simulink model "rasoc_tesis_v4"  (R2021a)
settings: Solver=FixedStepAuto  StartTime=0.0  StopTime=inf  FixedStep=0.01  RelTol=1e-3
values from neighbouring files (symbols this model uses):
  a = 0.445    [param_tesis.m]
  a_max = v_max/dt    (= 0.8)    [param_tesis.m]
  alt_z = 0    [param_tesis.m]
  B = 0.5    [param_tesis.m]
  currentPose = [47 43.5 0]    [param_tesis.m]
  efic_red = 0.95    [param_tesis.m]
  goalPose = [1.5 5 pi/2]    [param_tesis.m]
  gpsBasePose = [1 44]    [param_tesis.m]
  kb = 8.93*(3/(1000*pi))    (= 0.00852752185086)    [param_tesis.m]
  kt = 0.077*sqrt(2)*3    [param_tesis.m]
  L = 0.55    [param_tesis.m]
  m_uva = 0    [param_tesis.m]
  n = 16    [param_tesis.m]
  r = 0.125    [param_tesis.m]
  Ra = Vnom/Ipeak    (= 14.2857142857)    [param_tesis.m]
  Rp = Ra*20    (= 285.714285714)    [param_tesis.m]
  t_lpf = 1/200    (= 0.005)    [param_tesis.m]
  tau_max = 5    [param_tesis.m]
  v_max = 0.8    [param_tesis.m]
  Vnom = 310    [param_tesis.m]
  w_max = 0.5    [param_tesis.m]
  waypoints = [currentPose(1), currentPose(2) ... (first row only)    [AstarHybrid_fn.m]    (also in param_tesis.m = AstarHybrid_fn(currentPose, goalPose))
undefined symbols (not defined in the file or in its folder): angular, DiscIntNeverNeededParam, Earth, linear, startTheta, startX, startY, WGS84
libraries: ros2lib x10, simulink x5, mobileRoboticsTrainingLib x3, robotmobilelib x2, pid_lib x2, robotalgslib x2, aerolibtransform2 x2, dspstat3 x1
(part 1 of 2)
settings Model: PacingRate=0.500000  OrderedModelArguments=off  Creator=maxim  LastModifiedBy=maxim
settings DataIOCC: InspectSignalLogs=on
settings OptimizationCC: DefaultParameterBehavior=Inlined  EnhancedBackFolding=on  PassReuseOutputArgsAs=Individual arguments  ZeroExternalMemoryAtStartup=off  ZeroInternalMemoryAtStartup=off  MaxStackSize=64  OptimizeBlockOrder=speed  DifferentSizesBufferReuse=on  OptimizationCustomize=off  EfficientTunableParamExpr=on
settings DebuggingCC: ParameterTunabilityLossMsg=error  SFMachineParentedDataDiag=warning
settings SFSimCC: MATLABDynamicMemAlloc=off
settings RTWCC: SystemTargetFile=ert.tlc  TemplateMakefile=ert_default_tmf  Toolchain=Colcon Tools
settings CodeAppCC: ForceParamTrailComments=on  IgnoreCustomStorageClasses=off  OperatorAnnotations=on  SimulinkDataObjDesc=on  SFDataObjDesc=on  InsertBlockDesc=on
settings ERTTargetCC: RootIOFormat=Structure reference  ERTCustomFileTemplate=example_file_process.tlc

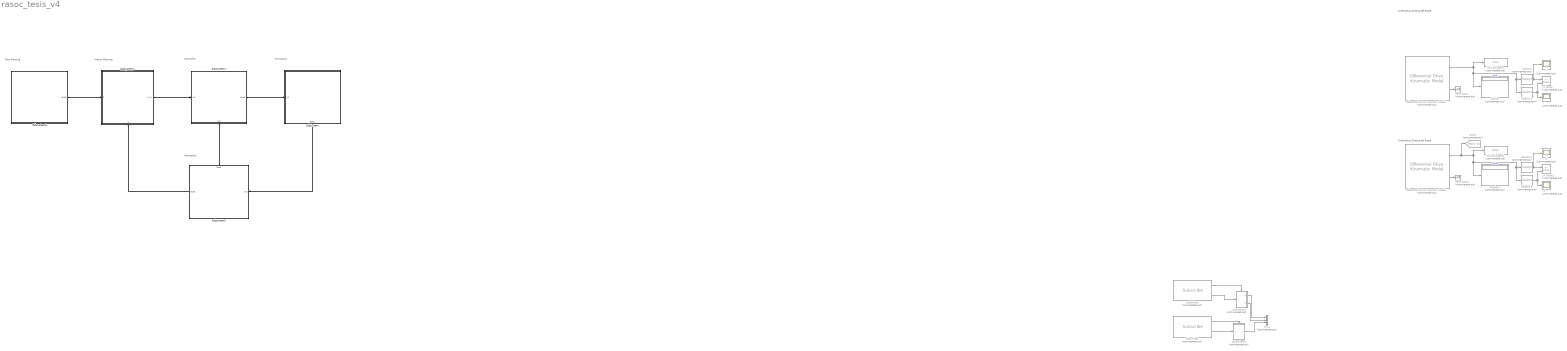
== system rasoc_tesis_v4 ==
  note: Cinemática Directa del Robot
  note: Motion Planning
  note: Controller
  note: Cinemática Directa del Robot
  note: Simulation
  note: Perception
  note: Path Planning
  Differential Drive Kinematic Model1 : robotmobilelib/Differential Drive Kinematic Model  Commented=on  VehicleInputs=Wheel Speeds  WheelRadius=r  WheelSpeedRange=[-inf inf]  TrackWidth=L  InitialState=[currentPose]'  SimulateUsing=Interpreted execution
      settings: SourceProductBaseCode=RO
  Differential Drive Kinematic Model2 : robotmobilelib/Differential Drive Kinematic Model  Commented=on  VehicleInputs=Vehicle Speed & Heading Angular Velocity  WheelRadius=r  WheelSpeedRange=[-inf inf]  TrackWidth=L  InitialState=[currentPose]'  SimulateUsing=Interpreted execution
      settings: SourceProductBaseCode=RO
  Display : Display  Commented=on
  Display1 : Display  Commented=on
  Goto4 : Goto  Commented=on  GotoTag=Pose_ros
  Mux1 : Mux  Commented=on  Inputs=3
  Selector : Selector  Commented=on  InputPortWidth=3  IndexOptions=Index vector (dialog)  Indices=[1]  OutputSizes=1
  Selector1 : Selector  Commented=on  InputPortWidth=3  IndexOptions=Index vector (dialog)  Indices=[2]  OutputSizes=1
  Selector2 : Selector  Commented=on  InputPortWidth=3  IndexOptions=Index vector (dialog)  Indices=[1]  OutputSizes=1
  Selector3 : Selector  Commented=on  InputPortWidth=3  IndexOptions=Index vector (dialog)  Indices=[2]  OutputSizes=1
  Subscribe1 : ros2lib/Subscribe  Commented=on  topicSource=Select from ROS network  topic=/odom  messageType=nav_msgs/Odometry  sampleTime=-1  QOSHistory=Keep last  QOSDepth=1  QOSReliability=Reliable  QOSDurability=Volatile
      settings: SourceProductBaseCode=RR
  Subscribe2 : ros2lib/Subscribe  Commented=on  topicSource=Select from ROS network  topic=/imu  messageType=sensor_msgs/Imu  sampleTime=-1  QOSHistory=Keep last  QOSDepth=1  QOSReliability=Reliable  QOSDurability=Volatile
      settings: SourceProductBaseCode=RR
  Subsystem : Subsystem
      settings: PortSchema="{\"entries\":[{\"content\":{\"sides\":[{\"content\":{\"connectorIds\":[\"In1\"]},\"type\":\"ConnectorPlacement.EquallySpacedRectSide\",\"uuid\":\"273e7eb3-3d1c-4843-aace-07e5779ada44\"},{\"content\":{\"connectorIds\":[],\"side\":\"RIGHT\"},\"type\":\"ConnectorPlacement.EquallySpacedRectSide\",\"uuid\":\"0ce8f36d-1762-4e21-817b-fb4bacc71d23\"},{\"content\":{\"connectorIds\":[],\"side\":\"TOP\"},\"type\":\"ConnectorPlacement.EquallySpacedRectSide\",\"uuid\":\"ca3ae62e-f410-42bb-944a-1dc9a9a102f7\"},{\"content\":{\"connectorIds\":[\"Out1\"],\"side\":\"BOTTOM\"},\"type\":\"ConnectorPlacement.EquallySpacedRectSide\",\"uuid\":\"b5aea1c3-8e14-4876-abba-3cc2b9e42095\"}]},\"type\":\"ConnectorPlacement.EquallySpacedConnector\",\"uuid\":\"a568fb3c-eb3c-49ee-882f-7e9a9c244b7d\"}],\"packageUris\":[\"http://schema.mathworks.com/mf0/Connector/R2020b\"],\"version\":\"1.0\"}"
      mask Display: image('$imagefile'); % Use "Edit Image" on toolstrip to change.
  Subsystem1 : Subsystem
      settings: PortSchema="{\"entries\":[{\"content\":{\"sides\":[{\"content\":{\"connectorIds\":[\"In1\"]},\"type\":\"ConnectorPlacement.EquallySpacedRectSide\",\"uuid\":\"7cc506d6-0df9-4dcf-87be-1a8fc33368cf\"},{\"content\":{\"connectorIds\":[\"Out1\"],\"side\":\"RIGHT\"},\"type\":\"ConnectorPlacement.EquallySpacedRectSide\",\"uuid\":\"9bee288a-7334-4d77-9b50-8b8395b9bab7\"},{\"content\":{\"connectorIds\":[],\"side\":\"TOP\"},\"type\":\"ConnectorPlacement.EquallySpacedRectSide\",\"uuid\":\"546aa84f-61a2-494c-9877-240dac3c06f9\"},{\"content\":{\"connectorIds\":[\"In2\"],\"side\":\"BOTTOM\"},\"type\":\"ConnectorPlacement.EquallySpacedRectSide\",\"uuid\":\"7e0fe68b-13b1-4e4e-82a9-96ee51fb6404\"}]},\"type\":\"ConnectorPlacement.EquallySpacedConnector\",\"uuid\":\"3eddb344-86cd-457c-a24d-297fc14890b0\"}],\"packageUris\":[\"http://schema.mathworks.com/mf0/Connector/R2020b\"],\"version\":\"1.0\"}"
      mask Display: image('$imagefile'); % Use "Edit Image" on toolstrip to change.
  Subsystem2 : Subsystem  Commented=on
  Subsystem3 : Subsystem  Commented=on
  Subsystem4 : Subsystem
      settings: PortSchema="{\"entries\":[{\"content\":{\"sides\":[{\"content\":{\"connectorIds\":[\"In1\"]},\"type\":\"ConnectorPlacement.EquallySpacedRectSide\",\"uuid\":\"4026ad61-f4ec-4a91-9be9-057f2d314736\"},{\"content\":{\"connectorIds\":[\"Out1\"],\"side\":\"RIGHT\"},\"type\":\"ConnectorPlacement.EquallySpacedRectSide\",\"uuid\":\"7c96fecf-2a17-4edc-9dde-8c00b1d53d18\"},{\"content\":{\"connectorIds\":[],\"side\":\"TOP\"},\"type\":\"ConnectorPlacement.EquallySpacedRectSide\",\"uuid\":\"976d1fbd-e5db-4716-a28c-2d13b9cfe893\"},{\"content\":{\"connectorIds\":[\"In2\"],\"side\":\"BOTTOM\"},\"type\":\"ConnectorPlacement.EquallySpacedRectSide\",\"uuid\":\"ea9d66a8-6726-4d07-bc02-8beb6f695a87\"}]},\"type\":\"ConnectorPlacement.EquallySpacedConnector\",\"uuid\":\"2f53d576-4576-48b6-bcca-625d1da1addb\"}],\"packageUris\":[\"http://schema.mathworks.com/mf0/Connector/R2020b\"],\"version\":\"1.0\"}"
      mask Display: image('$imagefile'); % Use "Edit Image" on toolstrip to change.
  Subsystem5 : Subsystem
      settings: PortSchema="{\"entries\":[{\"content\":{\"sides\":[{\"content\":{\"connectorIds\":[\"Out2\"]},\"type\":\"ConnectorPlacement.EquallySpacedRectSide\",\"uuid\":\"c37bb481-eb7e-4f76-88a9-7f2083741892\"},{\"content\":{\"connectorIds\":[\"In1\"],\"side\":\"RIGHT\"},\"type\":\"ConnectorPlacement.EquallySpacedRectSide\",\"uuid\":\"486068a6-059f-443b-b346-93df6811aae6\"},{\"content\":{\"connectorIds\":[\"Out1\"],\"side\":\"TOP\"},\"type\":\"ConnectorPlacement.EquallySpacedRectSide\",\"uuid\":\"f054f05a-6c52-4114-8c0f-0faeb4030005\"}]},\"type\":\"ConnectorPlacement.EquallySpacedConnector\",\"uuid\":\"e0be5d63-417f-4805-bb33-2fed0a69e720\"}],\"packageUris\":[\"http://schema.mathworks.com/mf0/Connector/R2020b\"],\"version\":\"1.0\"}"
      mask Display: image('$imagefile'); % Use "Edit Image" on toolstrip to change.
  Subsystem6 : Subsystem
      mask Display: image('$imagefile'); % Use "Edit Image" on toolstrip to change.
  Terminator : Terminator  Commented=on
  Terminator1 : Terminator  Commented=on
  To Workspace : ToWorkspace  Commented=on  VariableName=Pose  SampleTime=-1
  To Workspace1 : ToWorkspace  Commented=on  VariableName=Pose1  SampleTime=-1
  XY Graph : simulink/Sinks/XY Graph  Commented=on  xmin=0  xmax=50  ymin=-5  ymax=40  st=-1
  XY Graph1 : simulink/Sinks/XY Graph  Commented=on  xmin=0  xmax=25  ymin=0  ymax=25  st=-1
  x : Scope  Commented=on
  x1 : Scope  Commented=on
  y : Scope  Commented=on
  y1 : Scope  Commented=on
  wires:
  Differential Drive Kinematic Model1/1 -> To Workspace/1, Selector1/1, Selector/1, Display/1  "state"
  Selector1/1 -> y/1, XY Graph/2
  Selector/1 -> x/1, XY Graph/1
  Differential Drive Kinematic Model1/2 -> Terminator/1
  Differential Drive Kinematic Model2/2 -> Terminator1/1
  Selector2/1 -> XY Graph1/1, x1/1
  Selector3/1 -> XY Graph1/2, y1/1
  Differential Drive Kinematic Model2/1 -> Goto4/1, Display1/1, Selector2/1, Selector3/1, To Workspace1/1  "state"
  Subsystem2/1(x_ros) -> Mux1/1
  Subscribe2/1 -> Subsystem3/Enable
  Subscribe1/1 -> Subsystem2/Enable
  Subscribe1/2 -> Subsystem2/1(In1)
  Subsystem2/2(y_ros) -> Mux1/2
  Subsystem3/1(angZ_ros) -> Mux1/3
  Subscribe2/2 -> Subsystem3/1(In1)
  Subsystem4/1(v* w*) -> Subsystem1/1(In1)
  Subsystem1/1(Out1) -> Subsystem/1(In1)
  Subsystem/1(Out1) -> Subsystem5/1(In1)
  Subsystem5/2(Out1) -> Subsystem4/2(2)
  Subsystem6/1(Out1) -> Subsystem4/1(1)
  Subsystem5/1(Out2) -> Subsystem1/2(In2)

== system rasoc_tesis_v4/Subsystem ==
  note: wL
  note: wR
  In1 : Inport
  Bus Selector1 : BusSelector  OutputSignals=wL,wR
  OutputROSGazebo : Subsystem
  Out1 : Outport
  wires:
  [newMsg] -> OutputROSGazebo/Enable
  Bus Selector1/2 -> OutputROSGazebo/3(wR)  "<wR>"
  [atGoal] -> OutputROSGazebo/1(atGoal)
  Bus Selector1/1 -> OutputROSGazebo/2(wL)  "<wL>"
  In1/1 -> Bus Selector1/1

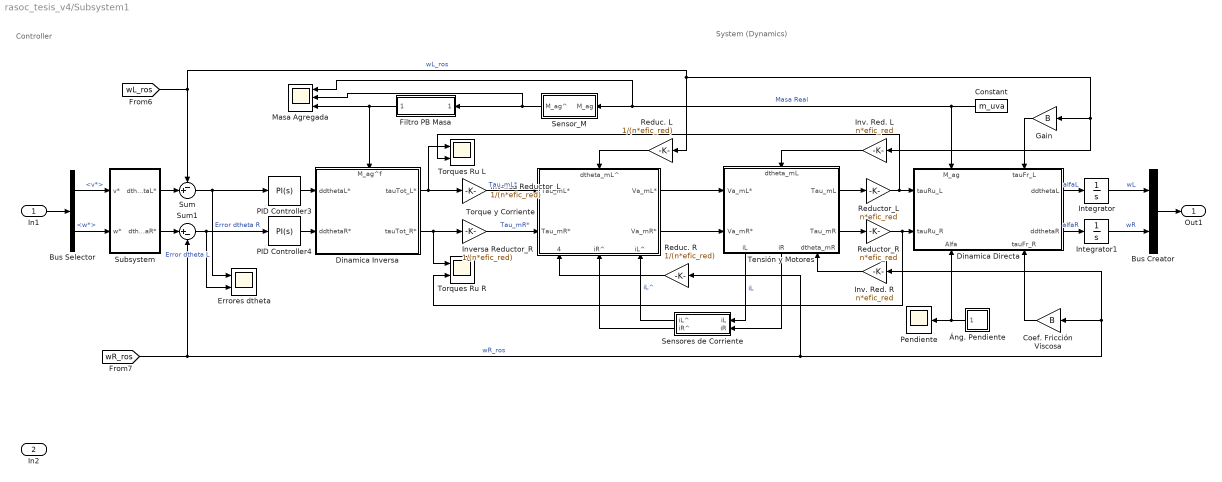
== system rasoc_tesis_v4/Subsystem1 ==
  note: Controller
  note: System (Dynamics)
  In1 : Inport
  In2 : Inport  Port=2
  Bus Creator : BusCreator  Inputs=2
  Bus Selector : BusSelector  OutputSignals=v*,w*
  Coef. Fricción Viscosa : Gain  Gain=B
  Constant : Constant  Value=m_uva
  Dinamica Directa : Subsystem
      settings: PortSchema="{\"entries\":[{\"content\":{\"sides\":[{\"content\":{\"connectorIds\":[\"In1\",\"In2\"]},\"type\":\"ConnectorPlacement.EquallySpacedRectSide\",\"uuid\":\"7724baec-8741-4c83-ab66-71b62264b439\"},{\"content\":{\"connectorIds\":[\"Out1\",\"Out2\"],\"side\":\"RIGHT\"},\"type\":\"ConnectorPlacement.EquallySpacedRectSide\",\"uuid\":\"83de1d79-8442-4360-ae36-8e267c42d9e7\"},{\"content\":{\"connectorIds\":[\"In3\",\"In4\"],\"side\":\"TOP\"},\"type\":\"ConnectorPlacement.EquallySpacedRectSide\",\"uuid\":\"5aa5624d-c3b7-443e-8b1c-4062683451e9\"},{\"content\":{\"connectorIds\":[\"In5\",\"In6\"],\"side\":\"BOTTOM\"},\"type\":\"ConnectorPlacement.EquallySpacedRectSide\",\"uuid\":\"38a03690-6302-43f4-ab4b-44458b1dd3d1\"}]},\"type\":\"ConnectorPlacement.EquallySpacedConnector\",\"uuid\":\"796ba574-cbe1-4118-90ae-27198d609312\"}],\"packageUris\":[\"http://schema.mathworks.com/mf0/Connector/R2020b\"],\"version\":\"1.0\"}"
  Dinamica Inversa : Subsystem
      settings: PortSchema="{\"entries\":[{\"content\":{\"sides\":[{\"content\":{\"connectorIds\":[\"In1\",\"In2\"]},\"type\":\"ConnectorPlacement.EquallySpacedRectSide\",\"uuid\":\"0faee1a4-a132-48bd-bc38-20a06c869d2e\"},{\"content\":{\"connectorIds\":[\"Out1\",\"Out2\"],\"side\":\"RIGHT\"},\"type\":\"ConnectorPlacement.EquallySpacedRectSide\",\"uuid\":\"c1af3771-28d7-4ef6-a87a-ceeaee1edff6\"},{\"content\":{\"connectorIds\":[\"In3\"],\"side\":\"TOP\"},\"type\":\"ConnectorPlacement.EquallySpacedRectSide\",\"uuid\":\"b4509dad-c3f6-4e9a-919d-cf82e4bac41d\"}]},\"type\":\"ConnectorPlacement.EquallySpacedConnector\",\"uuid\":\"1e7b5fad-e8ed-45a7-be76-1d23f7a948ab\"}],\"packageUris\":[\"http://schema.mathworks.com/mf0/Connector/R2020b\"],\"version\":\"1.0\"}"
  Errores dtheta : Scope  NumInputPorts=2
  Filtro PB Masa : Subsystem
  Gain : Gain  Gain=B
  Integrator : Integrator
  Integrator1 : Integrator
  Inv. Red. L : Gain  Gain=n*efic_red
  Inv. Red. R : Gain  Gain=n*efic_red
  Inversa Reductor_L : Gain  Gain=1/(n*efic_red)
  Inversa Reductor_R : Gain  Gain=1/(n*efic_red)
  Masa Agregada : Scope  NumInputPorts=3
  PID Controller3 : pid_lib/PID Controller  Controller=PI  Form=Parallel  TimeDomain=Continuous-time  UseExternalTs=off  SampleTime=-1  IntegratorMethod=Forward Euler  FilterMethod=Forward Euler  ControllerParametersSource=internal  P=56.2149208018988  I=55.3182760647861  D=2.6204  UseFilter=on  N=1661.0164  TunerSelectOption=Transfer Function Based (PID Tuner App)  InitialConditionSource=internal  InitialConditionForIntegrator=0  InitialConditionForFilter=0  DifferentiatorICPrevScaledInput=0  ExternalReset=none  TrackingMode=off  Kt=1  LimitOutput=off  SatLimitsSource=internal  UpperSaturationLimit=inf  LowerSaturationLimit=-inf  LinearizeAsGain=on  AntiWindupMode=none  Kb=1  POutMin=[]  POutMax=[]  IOutMin=[]  IOutMax=[]  DOutMin=[]  DOutMax=[]  NOutMin=[]  NOutMax=[]  SumOutMin=[]  SumOutMax=[]  SaturationOutMin=[]  SaturationOutMax=[]  PParamMin=[]  PParamMax=[]  IParamMin=[]  IParamMax=[]  DParamMin=[]  DParamMax=[]  NParamMin=[]  NParamMax=[]  KbParamMin=[]  KbParamMax=[]  KtParamMin=[]  KtParamMax=[]  KbOutMin=[]  KbOutMax=[]  KtOutMin=[]  KtOutMax=[]  IntegratorOutMin=[]  IntegratorOutMax=[]  FilterOutMin=[]  FilterOutMax=[]  SumI1OutMin=[]  SumI1OutMax=[]  SumI2OutMin=[]  SumI2OutMax=[]  SumI3OutMin=[]  SumI3OutMax=[]  SumI4OutMin=[]  SumI4OutMax=[]  SumDOutMin=[]  SumDOutMax=[]  DifferentiatorOutMin=[]  DifferentiatorOutMax=[]  FilterDiffOutCoefMin=[]  FilterDiffOutCoefMax=[]  ReciprocalOutMin=[]  ReciprocalOutMax=[]  SumDenOutMin=[]  SumDenOutMax=[]  SumNumOutMin=[]  SumNumOutMax=[]  DivideOutMin=[]  DivideOutMax=[]  UdiffTsProdOutMin=[]  UdiffTsProdOutMax=[]  NTsProdOutMin=[]  NTsProdOutMax=[]  UintegralTsProdOutMin=[]  UintegralTsProdOutMax=[]  UngainTsProdOutMin=[]  UngainTsProdOutMax=[]  IntegratorContinuousStateAttributes=''  IntegratorStateMustResolveToSignalObject=off  IntegratorRTWStateStorageClass=Auto  FilterContinuousStateAttributes=''  FilterStateMustResolveToSignalObject=off  FilterRTWStateStorageClass=Auto  ParallelPVariant=InternalParameters  IdealPVariant=Disabled  IVariant=InternalParameters  DVariant=Disabled  IntegratorVariant=Continuous  SatVariant=Disabled  AWVariant=Passthrough  PCopyVariant=Disabled  TRVariant=Disabled  FdbkBlocksVariant=Forward  IdealPFdbkVariant=Disabled  SatFdbkVariant=Disabled  DerivativeFilterVariant=Disabled  NVariant=Disabled  NCopyVariant=Disabled_SignalSpec  FilterICVariant=Disabled  IntegratorICVariant=InternalICs  ExternalResetVariant=Disabled  TRSumVariant=Passthrough  SumFdbkVariant=Disabled  SumVariant=Sum_PI  TsampFilterVariant=InternalTs  TsampNgainVariant=Passthrough  TsampIntegralVariant=Passthrough  ExternalSaturationOutDataTypeStr=Inherit: Same as second input
  PID Controller4 : pid_lib/PID Controller  Controller=PI  Form=Parallel  TimeDomain=Continuous-time  UseExternalTs=off  SampleTime=-1  IntegratorMethod=Forward Euler  FilterMethod=Forward Euler  ControllerParametersSource=internal  P=56.2149208018988  I=55.3182760647861  D=2.6204  UseFilter=on  N=1661.0164  TunerSelectOption=Transfer Function Based (PID Tuner App)  InitialConditionSource=internal  InitialConditionForIntegrator=0  InitialConditionForFilter=0  DifferentiatorICPrevScaledInput=0  ExternalReset=none  TrackingMode=off  Kt=1  LimitOutput=off  SatLimitsSource=internal  UpperSaturationLimit=inf  LowerSaturationLimit=-inf  LinearizeAsGain=on  AntiWindupMode=none  Kb=1  POutMin=[]  POutMax=[]  IOutMin=[]  IOutMax=[]  DOutMin=[]  DOutMax=[]  NOutMin=[]  NOutMax=[]  SumOutMin=[]  SumOutMax=[]  SaturationOutMin=[]  SaturationOutMax=[]  PParamMin=[]  PParamMax=[]  IParamMin=[]  IParamMax=[]  DParamMin=[]  DParamMax=[]  NParamMin=[]  NParamMax=[]  KbParamMin=[]  KbParamMax=[]  KtParamMin=[]  KtParamMax=[]  KbOutMin=[]  KbOutMax=[]  KtOutMin=[]  KtOutMax=[]  IntegratorOutMin=[]  IntegratorOutMax=[]  FilterOutMin=[]  FilterOutMax=[]  SumI1OutMin=[]  SumI1OutMax=[]  SumI2OutMin=[]  SumI2OutMax=[]  SumI3OutMin=[]  SumI3OutMax=[]  SumI4OutMin=[]  SumI4OutMax=[]  SumDOutMin=[]  SumDOutMax=[]  DifferentiatorOutMin=[]  DifferentiatorOutMax=[]  FilterDiffOutCoefMin=[]  FilterDiffOutCoefMax=[]  ReciprocalOutMin=[]  ReciprocalOutMax=[]  SumDenOutMin=[]  SumDenOutMax=[]  SumNumOutMin=[]  SumNumOutMax=[]  DivideOutMin=[]  DivideOutMax=[]  UdiffTsProdOutMin=[]  UdiffTsProdOutMax=[]  NTsProdOutMin=[]  NTsProdOutMax=[]  UintegralTsProdOutMin=[]  UintegralTsProdOutMax=[]  UngainTsProdOutMin=[]  UngainTsProdOutMax=[]  IntegratorContinuousStateAttributes=''  IntegratorStateMustResolveToSignalObject=off  IntegratorRTWStateStorageClass=Auto  FilterContinuousStateAttributes=''  FilterStateMustResolveToSignalObject=off  FilterRTWStateStorageClass=Auto  ParallelPVariant=InternalParameters  IdealPVariant=Disabled  IVariant=InternalParameters  DVariant=Disabled  IntegratorVariant=Continuous  SatVariant=Disabled  AWVariant=Passthrough  PCopyVariant=Disabled  TRVariant=Disabled  FdbkBlocksVariant=Forward  IdealPFdbkVariant=Disabled  SatFdbkVariant=Disabled  DerivativeFilterVariant=Disabled  NVariant=Disabled  NCopyVariant=Disabled_SignalSpec  FilterICVariant=Disabled  IntegratorICVariant=InternalICs  ExternalResetVariant=Disabled  TRSumVariant=Passthrough  SumFdbkVariant=Disabled  SumVariant=Sum_PI  TsampFilterVariant=InternalTs  TsampNgainVariant=Passthrough  TsampIntegralVariant=Passthrough  ExternalSaturationOutDataTypeStr=Inherit: Same as second input
  Pendiente : Scope
  Reduc. L : Gain  Gain=1/(n*efic_red)
  Reduc. R : Gain  Gain=1/(n*efic_red)
  Reductor_L : Gain  Gain=n*efic_red
  Reductor_R : Gain  Gain=n*efic_red
  Sensor_M : Subsystem
  Sensores de Corriente : Subsystem
  Subsystem : Subsystem
  Sum : Sum  Inputs=-+|
  Sum1 : Sum  Inputs=|+-
  Tensión y Motores : Subsystem
      settings: PortSchema="{\"entries\":[{\"content\":{\"sides\":[{\"content\":{\"connectorIds\":[\"In1\",\"In2\"]},\"type\":\"ConnectorPlacement.EquallySpacedRectSide\",\"uuid\":\"3ebe32f1-671c-48b5-a96d-67422499d9d8\"},{\"content\":{\"connectorIds\":[\"Out1\",\"Out2\"],\"side\":\"RIGHT\"},\"type\":\"ConnectorPlacement.EquallySpacedRectSide\",\"uuid\":\"07bd6e19-f9f7-4708-a097-3a0981aaf918\"},{\"content\":{\"connectorIds\":[\"In3\"],\"side\":\"TOP\"},\"type\":\"ConnectorPlacement.EquallySpacedRectSide\",\"uuid\":\"1235efa7-89af-450e-95aa-661cc319100f\"},{\"content\":{\"connectorIds\":[\"Out3\",\"Out4\",\"In4\"],\"side\":\"BOTTOM\"},\"type\":\"ConnectorPlacement.EquallySpacedRectSide\",\"uuid\":\"fc8cd9db-5607-4c14-9128-657f9a69419b\"}]},\"type\":\"ConnectorPlacement.EquallySpacedConnector\",\"uuid\":\"dbd94f6a-853e-4e3f-aaf2-5cf0eb955b89\"}],\"packageUris\":[\"http://schema.mathworks.com/mf0/Connector/R2020b\"],\"version\":\"1.0\"}"
  Torque y Corriente : Subsystem
      settings: PortSchema="{\"entries\":[{\"content\":{\"sides\":[{\"content\":{\"connectorIds\":[\"In1\",\"In2\"]},\"type\":\"ConnectorPlacement.EquallySpacedRectSide\",\"uuid\":\"fc3b99ab-82cb-4435-a104-343013dc5d5c\"},{\"content\":{\"connectorIds\":[\"Out1\",\"Out2\"],\"side\":\"RIGHT\"},\"type\":\"ConnectorPlacement.EquallySpacedRectSide\",\"uuid\":\"5ceb6380-9217-497c-9055-30e7b1371d6a\"},{\"content\":{\"connectorIds\":[\"In3\"],\"side\":\"TOP\"},\"type\":\"ConnectorPlacement.EquallySpacedRectSide\",\"uuid\":\"8bd5d57e-4a77-4e38-967f-f45b906ed799\"},{\"content\":{\"connectorIds\":[\"In4\",\"In5\",\"In6\"],\"side\":\"BOTTOM\"},\"type\":\"ConnectorPlacement.EquallySpacedRectSide\",\"uuid\":\"e6ffd4bd-cc9d-403e-b7b7-7878d8809b18\"}]},\"type\":\"ConnectorPlacement.EquallySpacedConnector\",\"uuid\":\"43fbc2ad-06f3-4e3b-a0a5-ad5db7ad1ee7\"}],\"packageUris\":[\"http://schema.mathworks.com/mf0/Connector/R2020b\"],\"version\":\"1.0\"}"
  Torques Ru L : Scope  NumInputPorts=2
  Torques Ru R : Scope  NumInputPorts=2
  Áng. Pendiente : Subsystem
  Out1 : Outport
  wires:
  Tensión y Motores/1(Tau_mL) -> Reductor_L/1
  Bus Selector/2 -> Subsystem/2(w*)  "<w*>"
  Subsystem/1(dthetaL*) -> Sum/2
  Tensión y Motores/4(iR) -> Sensores de Corriente/2(iR)
  Dinamica Inversa/1(tauTot_L*) -> Inversa Reductor_L/1, Torques Ru L/1
  In1/1 -> Bus Selector/1
  [wR_ros] -> Inv. Red. R/1, Coef. Fricción Viscosa/1, Reduc. R/1, Sum1/2  "wR_ros"
  Reduc. R/1 -> Torque y Corriente/4(dtheta_mR^)
  Gain/1 -> Dinamica Directa/4(tauFr_L)
  Inv. Red. R/1 -> Tensión y Motores/4(dtheta_mR)
  Sensor_M/1(M_ag^) -> Masa Agregada/2, Filtro PB Masa/1(M_ag^)
  Inversa Reductor_R/1 -> Torque y Corriente/2(Tau_mR*)  "Tau_mR*"
  Sensores de Corriente/1(iL^) -> Torque y Corriente/6(iL^)  "iL^"
  Dinamica Inversa/2(tauTot_R*) -> Torques Ru R/1, Inversa Reductor_R/1
  Sum/1 -> Errores dtheta/1, PID Controller3/1  "Error dtheta L"
  Dinamica Directa/1(ddthetaL) -> Integrator/1  "alfaL"
  Reductor_L/1 -> Torques Ru L/2, Dinamica Directa/1(tauRu_L)
  PID Controller4/1 -> Dinamica Inversa/2(ddthetaR*)
  Torque y Corriente/2(Va_mR*) -> Tensión y Motores/2(Va_mR*)
  [wL_ros] -> Reduc. L/1, Gain/1, Inv. Red. L/1, Sum/1  "wL_ros"
  Bus Creator/1 -> Out1/1
  Áng. Pendiente/1(Alfa) -> Pendiente/1, Dinamica Directa/5(Alfa)
  Sensores de Corriente/2(iR^) -> Torque y Corriente/5(iR^)
  Tensión y Motores/2(Tau_mR) -> Reductor_R/1
  PID Controller3/1 -> Dinamica Inversa/1(ddthetaL*)
  Tensión y Motores/3(iL) -> Sensores de Corriente/1(iL)  "iL"
  Coef. Fricción Viscosa/1 -> Dinamica Directa/6(tauFr_R)
  Inv. Red. L/1 -> Tensión y Motores/3(dtheta_mL)
  Sum1/1 -> Errores dtheta/2, PID Controller4/1  "Error dtheta R"
  Subsystem/2(dthetaR*) -> Sum1/1
  Inversa Reductor_L/1 -> Torque y Corriente/1(Tau_mL*)  "Tau_mL*"
  Filtro PB Masa/1(M_ag^f) -> Masa Agregada/3, Dinamica Inversa/3(M_ag^f)
  Constant/1 -> Dinamica Directa/3(M_ag), Masa Agregada/1, Sensor_M/1(M_ag)  "Masa Real"
  Reductor_R/1 -> Dinamica Directa/2(tauRu_R), Torques Ru R/2
  Reduc. L/1 -> Torque y Corriente/3(dtheta_mL^)
  Dinamica Directa/2(ddthetaR) -> Integrator1/1  "alfaR"
  Torque y Corriente/1(Va_mL*) -> Tensión y Motores/1(Va_mL*)
  Bus Selector/1 -> Subsystem/1(v*)  "<v*>"
  Integrator/1 -> Bus Creator/1  "wL"
  Integrator1/1 -> Bus Creator/2  "wR"

== system rasoc_tesis_v4/Subsystem2 ==
  In1 : Inport
  Enable : EnablePort
  Bus Selector : BusSelector  OutputSignals=pose.pose.position.x,pose.pose.position.y
  XY Graph2 : simulink/Sinks/XY Graph  xmin=-25  xmax=25  ymin=-25  ymax=25  st=-1
  x2 : Scope
  x_ros : Outport
  y_ros : Outport  Port=2
  wires:
  Bus Selector/1 -> x_ros/1, x2/1, XY Graph2/1  "<x>"
  In1/1 -> Bus Selector/1
  Bus Selector/2 -> y_ros/1, XY Graph2/2  "<y>"

== system rasoc_tesis_v4/Subsystem3 ==
  In1 : Inport
  Enable : EnablePort
  Bus Selector : BusSelector  OutputSignals=angular_velocity.z
  angZ_ros : Outport
  wires:
  In1/1 -> Bus Selector/1
  Bus Selector/1 -> angZ_ros/1  "<z>"

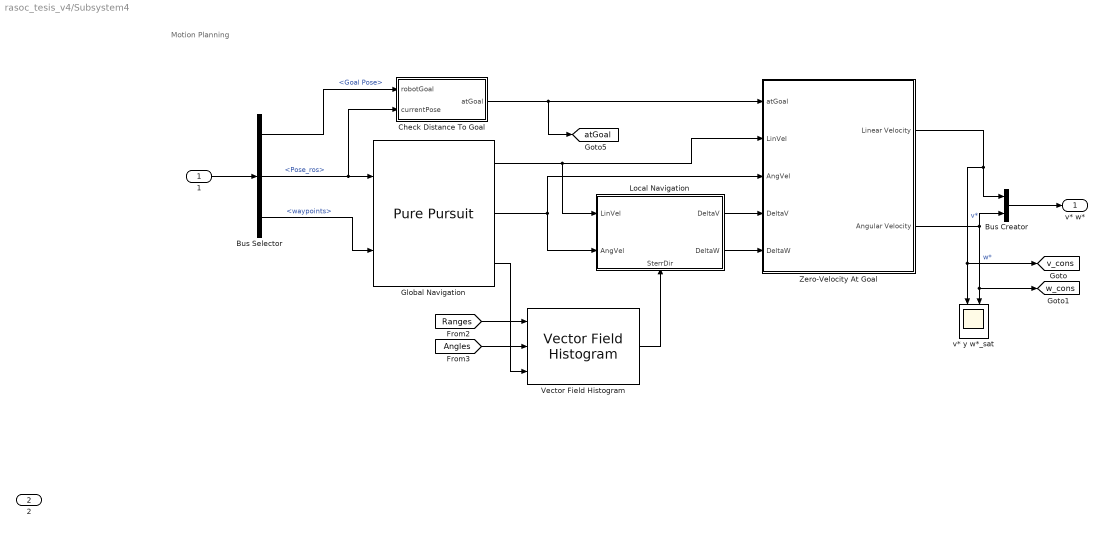
== system rasoc_tesis_v4/Subsystem4 ==
  note: Motion Planning
  1 : Inport
  2 : Inport  Port=2
  Bus Creator : BusCreator  Inputs=2
  Bus Selector : BusSelector  OutputSignals=Goal Pose,Pose_ros,waypoints
  Check Distance To Goal : Subsystem
  Global Navigation : robotalgslib/Pure Pursuit  DesiredLinearVelocity=v_max  MaxAngularVelocity=w_max  LookaheadDistance=1  TargetDirPort=on  SimulateUsing=Interpreted execution
  Local Navigation : Subsystem
      settings: PortSchema="{\"entries\":[{\"content\":{\"sides\":[{\"content\":{\"connectorIds\":[\"In1\",\"In2\"]},\"type\":\"ConnectorPlacement.EquallySpacedRectSide\",\"uuid\":\"55186746-5694-4bd2-a09a-d99615b0eaad\"},{\"content\":{\"connectorIds\":[\"Out1\",\"Out2\"],\"side\":\"RIGHT\"},\"type\":\"ConnectorPlacement.EquallySpacedRectSide\",\"uuid\":\"8ed27988-a77b-44ab-b7e0-da0854fe49ff\"},{\"content\":{\"connectorIds\":[],\"side\":\"TOP\"},\"type\":\"ConnectorPlacement.EquallySpacedRectSide\",\"uuid\":\"74002954-c61f-42a5-a263-bdcb6de94306\"},{\"content\":{\"connectorIds\":[\"In3\"],\"side\":\"BOTTOM\"},\"type\":\"ConnectorPlacement.EquallySpacedRectSide\",\"uuid\":\"d133e0cc-8222-4072-a760-f949dd9fd9b6\"}]},\"type\":\"ConnectorPlacement.EquallySpacedConnector\",\"uuid\":\"c719e9a2-6acd-4f9c-a46e-c9942eb848c4\"}],\"packageUris\":[\"http://schema.mathworks.com/mf0/Connector/R2020b\"],\"version\":\"1.0\"}"
  Vector Field Histogram : robotalgslib/Vector Field Histogram  NumAngularSectors=180  DistanceLimits=[ 0.06, 3 ]  HistogramThresholds=[ 3, 8 ]  RobotRadius=r  SafetyDistance=lidar_dist  MinTurningRadius=R  SimulateUsing=Interpreted execution  TargetDirectionWeight=5  CurrentDirectionWeight=2  PreviousDirectionWeight=2
      settings: SourceProductBaseCode=NV,RO
  Zero-Velocity At Goal : Subsystem
  v* y w*_sat : Scope  NumInputPorts=2
  v* w* : Outport
  tag scope: atGoal=global, v_cons=global, w_cons=global
  wires:
  Zero-Velocity At Goal/1(Linear Velocity) -> [v_cons], v* y w*_sat/1, Bus Creator/1  "v*"
  Global Navigation/1 -> Zero-Velocity At Goal/2(LinVel), Local Navigation/1(LinVel)
  Check Distance To Goal/1(atGoal) -> [atGoal], Zero-Velocity At Goal/1(atGoal)
  Bus Creator/1 -> v* w*/1
  Zero-Velocity At Goal/2(Angular Velocity) -> Bus Creator/2, [w_cons], v* y w*_sat/2  "w*"
  Vector Field Histogram/1 -> Local Navigation/3(SterrDir)
  [Ranges] -> Vector Field Histogram/1
  Global Navigation/2 -> Local Navigation/2(AngVel), Zero-Velocity At Goal/3(AngVel)
  Global Navigation/3 -> Vector Field Histogram/3
  Local Navigation/1(DeltaV) -> Zero-Velocity At Goal/4(DeltaV)
  Local Navigation/2(DeltaW) -> Zero-Velocity At Goal/5(DeltaW)
  Bus Selector/1 -> Check Distance To Goal/1(robotGoal)  "<Goal Pose>"
  Bus Selector/2 -> Check Distance To Goal/2(currentPose), Global Navigation/1  "<Pose_ros>"
  [Angles] -> Vector Field Histogram/2
  Bus Selector/3 -> Global Navigation/2  "<waypoints>"
  1/1 -> Bus Selector/1

== system rasoc_tesis_v4/Subsystem5 ==
  In1 : Inport
  InputROSGazebo : Subsystem
      settings: PortSchema="{\"entries\":[{\"content\":{\"sides\":[{\"content\":{\"connectorIds\":[]},\"type\":\"ConnectorPlacement.EquallySpacedRectSide\",\"uuid\":\"e5f26438-64a4-41f7-8cc6-3d189d8fc99d\"},{\"content\":{\"connectorIds\":[\"Out1\",\"Out2\",\"Out3\",\"Out4\",\"Out5\"],\"side\":\"RIGHT\"},\"type\":\"ConnectorPlacement.EquallySpacedRectSide\",\"uuid\":\"ad1152d5-f521-47db-b945-149d6bcc843b\"},{\"content\":{\"connectorIds\":[\"Out6\"],\"side\":\"TOP\"},\"type\":\"ConnectorPlacement.EquallySpacedRectSide\",\"uuid\":\"4f862710-1963-4fdd-a455-d6aa0cda1932\"}]},\"type\":\"ConnectorPlacement.EquallySpacedConnector\",\"uuid\":\"c0564360-50d0-4b81-ab53-7856385677dd\"}],\"packageUris\":[\"http://schema.mathworks.com/mf0/Connector/R2020b\"],\"version\":\"1.0\"}"
  Out2 : Outport
  Out1 : Outport  Port=2
  tag scope: Angles=global, Pose_ros=global, Ranges=global, newMsg=global, wL_ros=global, wR_ros=global
  wires:
  InputROSGazebo/2(Angles) -> [Angles]
  InputROSGazebo/1(Ranges) -> [Ranges]
  InputROSGazebo/3(Pose_ros) -> [Pose_ros]
  InputROSGazebo/6(NewMsg) -> [newMsg]
  InputROSGazebo/4(wL_ros) -> [wL_ros]
  InputROSGazebo/5(wR_ros) -> [wR_ros]

== system rasoc_tesis_v4/Subsystem6 ==
  " " : Constant  Value=waypoints
  Bus Creator : BusCreator  Inputs=3
  Goal Pose : Constant  Value=goalPose
  Out1 : Outport
  wires:
  Goal Pose/1 -> Bus Creator/1  "Goal Pose"
  " "/1 -> Bus Creator/3  "waypoints"
  [Pose_ros] -> Bus Creator/2  "Pose_ros"
  Bus Creator/1 -> Out1/1

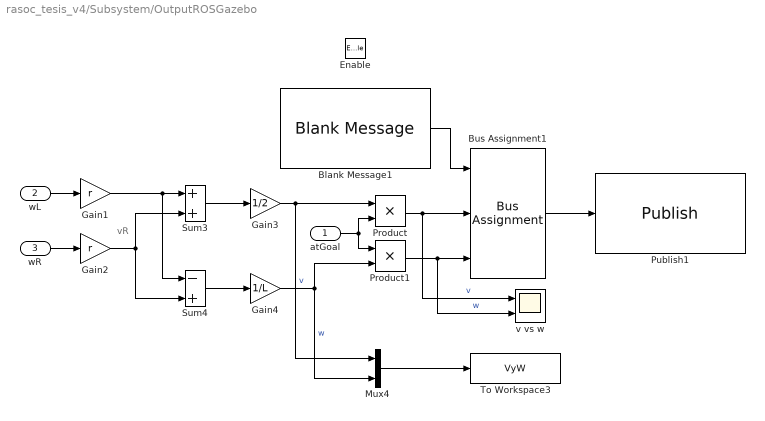
== system rasoc_tesis_v4/Subsystem/OutputROSGazebo ==
  note: vR
  atGoal : Inport
  wL : Inport  Port=2
  wR : Inport  Port=3
  Enable : EnablePort
  Blank Message1 : ros2lib/Blank Message  messageType=geometry_msgs/Twist  SampleTime=inf
      settings: SourceProductBaseCode=RR
  Bus Assignment1 : BusAssignment  AssignedSignals=linear.x,angular.z
  Gain1 : Gain  Gain=r
  Gain2 : Gain  Gain=r
  Gain3 : Gain  Gain=1/2
  Gain4 : Gain  Gain=1/L
  Mux4 : Mux  Inputs=2
  Product : Product
  Product1 : Product
  Publish1 : ros2lib/Publish  topicSource=Select from ROS network  topic=/demo/cmd_vel  messageType=geometry_msgs/Twist  QOSHistory=Keep last  QOSDepth=1  QOSReliability=Reliable  QOSDurability=Volatile
      settings: SourceProductBaseCode=RR
  Sum3 : Sum
  Sum4 : Sum  Inputs=-+
  To Workspace3 : ToWorkspace  VariableName=VyW  SampleTime=-1
  v vs w : Scope  NumInputPorts=2
  wires:
  Bus Assignment1/1 -> Publish1/1
  Blank Message1/1 -> Bus Assignment1/1
  Mux4/1 -> To Workspace3/1
  Gain2/1 -> Sum3/2, Sum4/2
  Gain1/1 -> Sum3/1, Sum4/1
  Sum3/1 -> Gain3/1
  Gain4/1 -> Product1/2, Mux4/2  "w"
  Gain3/1 -> Product/1, Mux4/1  "v"
  Sum4/1 -> Gain4/1
  wL/1 -> Gain1/1
  wR/1 -> Gain2/1
  atGoal/1 -> Product/2, Product1/1
  Product1/1 -> Bus Assignment1/3, v vs w/2  "w"
  Product/1 -> Bus Assignment1/2, v vs w/1  "v"

== system rasoc_tesis_v4/Subsystem1/Dinamica Directa ==
  tauRu_L : Inport
  tauRu_R : Inport  Port=2
  M_ag : Inport  Port=3
  tauFr_L : Inport  Port=4
  Alfa : Inport  Port=5
  tauFr_R : Inport  Port=6
  MATLAB Function : MATLAB Function  TreatAsAtomicUnit=on
  Mux : Mux  Inputs=2
  ddthetaL : Outport
  ddthetaR : Outport  Port=2
  wires:
  MATLAB Function/1(ddthetaL) -> ddthetaL/1
  MATLAB Function/2(ddthetaR) -> ddthetaR/1
  tauRu_R/1 -> MATLAB Function/2(tauRu_R)
  tauRu_L/1 -> MATLAB Function/1(tauRu_L)
  M_ag/1 -> MATLAB Function/3(M_ag)
  Mux/1 -> MATLAB Function/4(tauFr)
  tauFr_L/1 -> Mux/2
  tauFr_R/1 -> Mux/1
  Alfa/1 -> MATLAB Function/5(alfa)

== system rasoc_tesis_v4/Subsystem1/Dinamica Inversa ==
  ddthetaL* : Inport
  ddthetaR* : Inport  Port=2
  M_ag^f : Inport  Port=3
  MATLAB Function : MATLAB Function  TreatAsAtomicUnit=on
  tauTot_L* : Outport
  tauTot_R* : Outport  Port=2
  wires:
  MATLAB Function/2(tauTot_R) -> tauTot_R*/1
  MATLAB Function/1(tauTot_L) -> tauTot_L*/1
  M_ag^f/1 -> MATLAB Function/3(M_ag)
  ddthetaL*/1 -> MATLAB Function/1(ddthetaL)
  ddthetaR*/1 -> MATLAB Function/2(ddthetaR)

== system rasoc_tesis_v4/Subsystem1/Filtro PB Masa ==
  M_ag^ : Inport
  Filtro PB Lento : StateSpace  A=[-1/2]  B=[1]  C=[1/2]  D=[0]  InitialCondition=0
  M_ag^f : Outport
  wires:
  Filtro PB Lento/1 -> M_ag^f/1
  M_ag^/1 -> Filtro PB Lento/1

== system rasoc_tesis_v4/Subsystem1/Sensor_M ==
  M_ag : Inport
  Gain : Gain  Gain=1/10
  Resolución : Quantizer  QuantizationInterval=20/3000  LinearizeAsGain=off
  Retardo : UnitDelay  SampleTime=-1  HasFrameUpgradeWarning=on
  Ruido : RandomNumber  Variance=5  SampleTime=0.01
  Sum : Sum  Inputs=++|
  M_ag^ : Outport
  wires:
  Retardo/1 -> M_ag^/1
  Resolución/1 -> Retardo/1
  M_ag/1 -> Sum/2
  Ruido/1 -> Gain/1
  Sum/1 -> Resolución/1
  Gain/1 -> Sum/1

== system rasoc_tesis_v4/Subsystem1/Sensores de Corriente ==
  iL : Inport
  iR : Inport  Port=2
  " " : StateSpace  A=[-1/1000]  B=[1]  C=[1/1000]  D=[0]  InitialCondition=0
  Filtro PB 1° Orden : StateSpace  A=[-1/1000]  B=[1]  C=[1/1000]  D=[0]  InitialCondition=0
  Resolución : Quantizer  QuantizationInterval=0.01  LinearizeAsGain=off
  Resolución1 : Quantizer  QuantizationInterval=0.01  LinearizeAsGain=off
  Ret. : UnitDelay  SampleTime=-1  HasFrameUpgradeWarning=on
  Retardo : UnitDelay  SampleTime=-1  HasFrameUpgradeWarning=on
  iL^ : Outport
  iR^ : Outport  Port=2
  wires:
  Filtro PB 1° Orden/1 -> Resolución/1
  " "/1 -> Resolución1/1
  iL/1 -> Filtro PB 1° Orden/1
  iR/1 -> " "/1
  Retardo/1 -> iL^/1
  Ret./1 -> iR^/1
  Resolución/1 -> Retardo/1
  Resolución1/1 -> Ret./1

== system rasoc_tesis_v4/Subsystem1/Subsystem ==
  v* : Inport
  w* : Inport  Port=2
  Gain : Gain  Gain=L/2
  Gain1 : Gain  Gain=1/r
  Gain2 : Gain  Gain=1/r
  Sum : Sum  Inputs=|+-
  Sum1 : Sum  Inputs=|++
  dthetaL* : Outport
  dthetaR* : Outport  Port=2
  wires:
  v*/1 -> Sum/1, Sum1/2
  w*/1 -> Gain/1
  Gain/1 -> Sum1/1, Sum/2
  Sum/1 -> Gain1/1
  Gain1/1 -> dthetaL*/1
  Gain2/1 -> dthetaR*/1
  Sum1/1 -> Gain2/1

== system rasoc_tesis_v4/Subsystem1/Tensión y Motores ==
  Va_mL* : Inport
  Va_mR* : Inport  Port=2
  dtheta_mL : Inport  Port=3
  dtheta_mR : Inport  Port=4
  Modulador de Tensión : Subsystem
  Motores : Subsystem
      settings: PortSchema="{\"entries\":[{\"content\":{\"sides\":[{\"content\":{\"connectorIds\":[\"In1\",\"In2\"]},\"type\":\"ConnectorPlacement.EquallySpacedRectSide\",\"uuid\":\"3ebe32f1-671c-48b5-a96d-67422499d9d8\"},{\"content\":{\"connectorIds\":[\"Out1\",\"Out2\"],\"side\":\"RIGHT\"},\"type\":\"ConnectorPlacement.EquallySpacedRectSide\",\"uuid\":\"07bd6e19-f9f7-4708-a097-3a0981aaf918\"},{\"content\":{\"connectorIds\":[\"In3\",\"In4\"],\"side\":\"TOP\"},\"type\":\"ConnectorPlacement.EquallySpacedRectSide\",\"uuid\":\"1235efa7-89af-450e-95aa-661cc319100f\"},{\"content\":{\"connectorIds\":[\"Out3\",\"Out4\"],\"side\":\"BOTTOM\"},\"type\":\"ConnectorPlacement.EquallySpacedRectSide\",\"uuid\":\"2ce1a4f0-d2da-4181-81ee-614a7e1b7156\"}]},\"type\":\"ConnectorPlacement.EquallySpacedConnector\",\"uuid\":\"dbd94f6a-853e-4e3f-aaf2-5cf0eb955b89\"}],\"packageUris\":[\"http://schema.mathworks.com/mf0/Connector/R2020b\"],\"version\":\"1.0\"}"
  Tau_mL : Outport
  Tau_mR : Outport  Port=2
  iL : Outport  Port=3
  iR : Outport  Port=4
  wires:
  Motores/1(Tau_mL) -> Tau_mL/1
  Motores/2(Tau_mR) -> Tau_mR/1
  Modulador de Tensión/2(Va_mR) -> Motores/2(Va_mR)
  Modulador de Tensión/1(Va_mL) -> Motores/1(Va_mL)
  Va_mR*/1 -> Modulador de Tensión/2(Va_mR*)
  Va_mL*/1 -> Modulador de Tensión/1(Va_mL*)
  Motores/3(iL) -> iR/1
  Motores/4(iR) -> iL/1
  dtheta_mL/1 -> Motores/3(dtheta_mL)
  dtheta_mR/1 -> Motores/4(dtheta_mR)

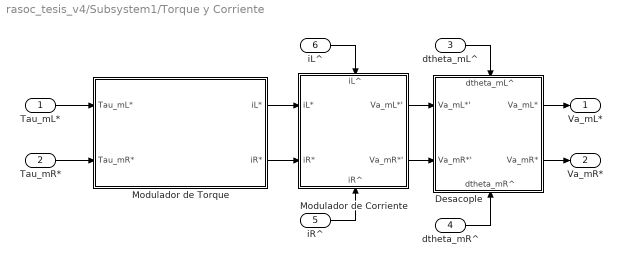
== system rasoc_tesis_v4/Subsystem1/Torque y Corriente ==
  Tau_mL* : Inport
  Tau_mR* : Inport  Port=2
  dtheta_mL^ : Inport  Port=3
  dtheta_mR^ : Inport  Port=4
  iR^ : Inport  Port=5
  iL^ : Inport  Port=6
  Desacople : Subsystem
      settings: PortSchema="{\"entries\":[{\"content\":{\"sides\":[{\"content\":{\"connectorIds\":[\"In1\",\"In2\"]},\"type\":\"ConnectorPlacement.EquallySpacedRectSide\",\"uuid\":\"3fca05c4-9944-4d1c-bfbf-1c7b323f5576\"},{\"content\":{\"connectorIds\":[\"Out1\",\"Out2\"],\"side\":\"RIGHT\"},\"type\":\"ConnectorPlacement.EquallySpacedRectSide\",\"uuid\":\"f7a735a9-0b51-4d0f-a212-abe97905570a\"},{\"content\":{\"connectorIds\":[\"In3\"],\"side\":\"TOP\"},\"type\":\"ConnectorPlacement.EquallySpacedRectSide\",\"uuid\":\"aeae328d-370b-49fe-a39a-1018b5d510af\"},{\"content\":{\"connectorIds\":[\"In4\"],\"side\":\"BOTTOM\"},\"type\":\"ConnectorPlacement.EquallySpacedRectSide\",\"uuid\":\"d29ba667-c237-4795-b87b-5386cf2b5124\"}]},\"type\":\"ConnectorPlacement.EquallySpacedConnector\",\"uuid\":\"90e38418-0668-4b70-a8ad-086f1cbc9972\"}],\"packageUris\":[\"http://schema.mathworks.com/mf0/Connector/R2020b\"],\"version\":\"1.0\"}"
  Modulador de Corriente : Subsystem
      settings: PortSchema="{\"entries\":[{\"content\":{\"sides\":[{\"content\":{\"connectorIds\":[\"In1\",\"In2\"]},\"type\":\"ConnectorPlacement.EquallySpacedRectSide\",\"uuid\":\"fa4e6480-e76c-4c1d-bc6f-319c8a12ca48\"},{\"content\":{\"connectorIds\":[\"Out1\",\"Out2\"],\"side\":\"RIGHT\"},\"type\":\"ConnectorPlacement.EquallySpacedRectSide\",\"uuid\":\"cb01f017-a7ce-4c54-8f9c-222b4f50ca72\"},{\"content\":{\"connectorIds\":[\"In3\"],\"side\":\"TOP\"},\"type\":\"ConnectorPlacement.EquallySpacedRectSide\",\"uuid\":\"6f59978a-ad4b-42f1-9161-9da3705aed1f\"},{\"content\":{\"connectorIds\":[\"In4\"],\"side\":\"BOTTOM\"},\"type\":\"ConnectorPlacement.EquallySpacedRectSide\",\"uuid\":\"3dae7d9a-d248-4757-9528-0813c3278129\"}]},\"type\":\"ConnectorPlacement.EquallySpacedConnector\",\"uuid\":\"a79a7fed-6874-41f4-b474-148d88d39a49\"}],\"packageUris\":[\"http://schema.mathworks.com/mf0/Connector/R2020b\"],\"version\":\"1.0\"}"
  Modulador de Torque : Subsystem
  Va_mL* : Outport
  Va_mR* : Outport  Port=2
  wires:
  dtheta_mL^/1 -> Desacople/3(dtheta_mL^)
  Tau_mR*/1 -> Modulador de Torque/2(Tau_mR*)
  Modulador de Torque/2(iR*) -> Modulador de Corriente/2(iR*)
  Modulador de Torque/1(iL*) -> Modulador de Corriente/1("iL* ")
  Tau_mL*/1 -> Modulador de Torque/1(Tau_mL*)
  iL^/1 -> Modulador de Corriente/3(iL^)
  iR^/1 -> Modulador de Corriente/4(iR^)
  Modulador de Corriente/1(Va_mL*') -> Desacople/1(Va_mL*')
  Modulador de Corriente/2(Va_mR*') -> Desacople/2(Va_mR*')
  Desacople/1(Va_mL*) -> Va_mL*/1
  Desacople/2(Va_mR*) -> Va_mR*/1
  dtheta_mR^/1 -> Desacople/4(dtheta_mR^)

== system rasoc_tesis_v4/Subsystem1/Áng. Pendiente ==
  Add : Sum  Inputs=++++
  Bajada : Step  Time=5  After=-30  SampleTime=0
  Plano Abajo : Step  Time=7  After=30  SampleTime=0
  Plano Arriba : Step  Time=4  After=-30  SampleTime=0
  Scope : Scope
  Subida : Step  Time=2  After=30  SampleTime=0
  Alfa : Outport
  wires:
  Add/1 -> Scope/1, Alfa/1
  Subida/1 -> Add/1
  Plano Arriba/1 -> Add/2
  Bajada/1 -> Add/3
  Plano Abajo/1 -> Add/4

== system rasoc_tesis_v4/Subsystem4/Check Distance To Goal ==
  note: Distance from Goal to satisfy that the robot has reached the goal
  robotGoal : Inport
  currentPose : Inport  Port=2
  Constant : Constant
  Dot Product : DotProduct  InputSameDT=on  OutDataTypeStr=Inherit: Inherit via internal rule
  Less Than : RelationalOperator  OutDataTypeStr=boolean  RndMeth=Simplest
  Selector : Selector  InputPortWidth=3  IndexOptions=Index vector (dialog)  Indices=[1 2]  OutputSizes=1
  Selector1 : Selector  InputPortWidth=3  IndexOptions=Index vector (dialog)  Indices=[1 2]  OutputSizes=1
  Sqrt : Sqrt  SaturateOnIntegerOverflow=on
  Subtract : Sum  Inputs=+-
  atGoal : Outport
  wires:
  robotGoal/1 -> Selector1/1
  Dot Product/1 -> Sqrt/1
  Constant/1 -> Less Than/2
  currentPose/1 -> Selector/1
  Less Than/1 -> atGoal/1
  Sqrt/1 -> Less Than/1
  Subtract/1 -> Dot Product/1, Dot Product/2
  Selector/1 -> Subtract/1
  Selector1/1 -> Subtract/2

== system rasoc_tesis_v4/Subsystem4/Local Navigation ==
  LinVel : Inport
  AngVel : Inport  Port=2
  SterrDir : Inport  Port=3
  If : If  IfExpression=u1 == 1
  Merge : Merge
  Merge1 : Merge
  Path Following : Subsystem  TreatAsAtomicUnit=on
  Recovery : Subsystem  TreatAsAtomicUnit=on
  Relational Operator : RelationalOperator  Operator=isNaN  OutDataTypeStr=boolean  RndMeth=Simplest
  DeltaV : Outport  VectorParamsAs1DForOutWhenUnconnected=off
  DeltaW : Outport  Port=2  VectorParamsAs1DForOutWhenUnconnected=off
  wires:
  Merge1/1 -> DeltaW/1
  LinVel/1 -> Recovery/1(LinVel)
  Recovery/1(dV) -> Merge/1
  Recovery/2(dW) -> Merge1/1
  Path Following/1(dV) -> Merge/2
  Path Following/2(dW) -> Merge1/2
  If/2 -> Path Following/Action
  Relational Operator/1 -> If/1
  SterrDir/1 -> Path Following/1(SteeringDirection), Relational Operator/1
  AngVel/1 -> Path Following/2(AngularVelocity), Recovery/2(AngVel)
  Merge/1 -> DeltaV/1
  If/1 -> Recovery/Action

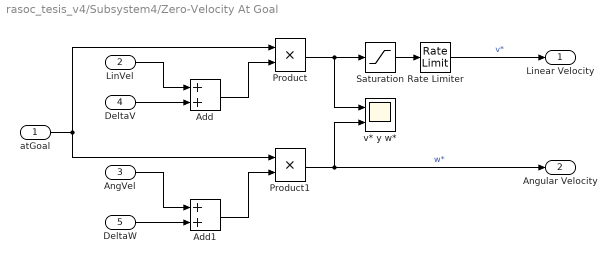
== system rasoc_tesis_v4/Subsystem4/Zero-Velocity At Goal ==
  atGoal : Inport
  LinVel : Inport  Port=2
  AngVel : Inport  Port=3
  DeltaV : Inport  Port=4
  DeltaW : Inport  Port=5
  Add : Sum
  Add1 : Sum
  Product : Product
  Product1 : Product
  Rate Limiter : RateLimiter  RisingSlewLimit=a_max  FallingSlewLimit=-a_max  SampleTimeMode=inherited
  Saturation : Saturate  UpperLimit=v_max  LowerLimit=-v_max
  v* y w* : Scope  NumInputPorts=2
  Linear Velocity : Outport  OutDataTypeStr=double
  Angular Velocity : Outport  Port=2  OutDataTypeStr=double
  wires:
  atGoal/1 -> Product/1, Product1/1
  AngVel/1 -> Add1/1
  LinVel/1 -> Add/1
  Add/1 -> Product/2
  DeltaV/1 -> Add/2
  Add1/1 -> Product1/2
  DeltaW/1 -> Add1/2
  Saturation/1 -> Rate Limiter/1
  Product1/1 -> v* y w*/2, Angular Velocity/1  "w*"
  Rate Limiter/1 -> Linear Velocity/1  "v*"
  Product/1 -> Saturation/1, v* y w*/1

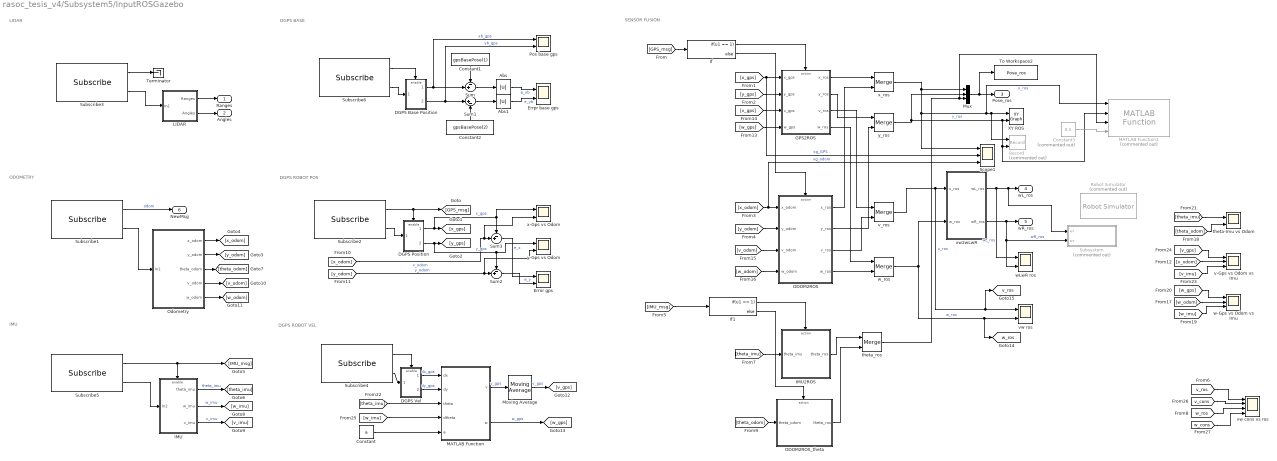
== system rasoc_tesis_v4/Subsystem5/InputROSGazebo ==
  note: DGPS BASE
  note: LIDAR
  note: ODOMETRY
  note: DGPS ROBOT POS
  note: IMU
  note: DGPS ROBOT VEL
  note: SENSOR FUSION
  Abs : Abs
  Abs1 : Abs
  Constant : Constant  Value=a
  Constant1 : Constant  Value=gpsBasePose(1)
  Constant2 : Constant  Value=gpsBasePose(2)
  Constant3 : Constant  Commented=on  Value=0.5
  DGPS Base Position : Subsystem
  DGPS Position : Subsystem
  DGPS Vel : Subsystem
  Error gps : Scope  NumInputPorts=2
  Errpr base gps : Scope  NumInputPorts=2
  GPS2ROS : Subsystem  TreatAsAtomicUnit=on
  IMU : Subsystem
  IMU2ROS : Subsystem  TreatAsAtomicUnit=on
  If : If  IfExpression=u1 == 1
  If1 : If  IfExpression=u1 == 1
  LIDAR : Subsystem
  MATLAB Function : MATLAB Function  TreatAsAtomicUnit=on
  MATLAB Function1 : mobileRoboticsTrainingLib/Robot Simulator/MATLAB Function  Commented=on  SystemSampleTime=-1  VariantActivationTime=update diagram  Latency=0  AutoFrameSizeCalculation=off
      settings: SourceProductName=Mobile Robotics Training Library
  Moving Average : dspstat3/Moving Average  Method=Sliding window  ForgettingFactorPort=off  SpecifyWindowLength=on  WindowLength=4  ForgettingFactor=0.9  SimulateUsing=Code generation
  Mux : Mux  Inputs=3
  ODOM2ROS : Subsystem  TreatAsAtomicUnit=on
  ODOM2ROS_theta : Subsystem  TreatAsAtomicUnit=on
  Odometry : Subsystem
  Pos base gps : Scope  NumInputPorts=2
  Record : Record  Commented=on  FileSettingsInternal="{\"entries\":[{\"content\":{\"excelSettings\":{\"content\":{},\"type\":\"Streamout.ExcelSettings\"}},\"type\":\"Streamout.FileSettingStorage\",\"uuid\":\"2701ad38-51b1-4612-8c68-417fbf51999a\"}],\"packageUris\":[\"http://schema.mathworks.com/mf0/streamout_blocks/R2020a\"],\"version\":\"1.0\"}"  Layout=[1 1]  SignalsInternal="{\"entries\":[{\"content\":{\"signals\":[{\"content\":{\"blockPath\":[\"rasoc_tesis_v4/Subsystem5/InputROSGazebo/Record\"],\"channel\":[],\"dimensions\":[1],\"domain\":\"rasoc_tesis_v4/subsystem5/inputrosgazebo/record\",\"lineColor\":\"#7e2f8e\",\"plots\":[1],\"port\":1,\"sid\":[\"\"],\"signalID\":28491,\"signalName\":\"x_ros\"},\"type\":\"RecordBlkView.Signal\",\"uuid\":\"86327079-759d-4581-b614-a804c86ae6c2\"},{\"content\":{\"blockPath\":[\"rasoc_tesis_v4/Subsystem5/InputROSGazebo/Record\"],\"channel\":[],\"dimensions\":[1],\"domain\":\"rasoc_tesis_v4/subsystem5/inputrosgazebo/record\",\"lineColor\":\"#7e2f8e\",\"plots\":[1],\"port\":2,\"sid\":[\"\"],\"signalID\":28495,\"signalName\":\"y_ros\"},\"type\":\"RecordBlkView.Signal\",\"uuid\":\"1a384cea-457b-4106-ad96-c112a79d26d3\"}]},\"type\":\"RecordBlkView.InputSignals\",\"uuid\":\"640b33bc-dbd8-4f70-99cc-05b3f9913783\"}],\"packageUris\":[\"http://schema.mathworks.com/mf0/streamout_blocks/R2020a\"],\"version\":\"1.0\"}"  VisualizationBindings="{\"xyplotplugin\":{\"info\":[{\"series\":[{\"bindingParametersList\":[{\"parameter\":\"X-Axis\",\"signalID\":28491,\"signalName\":\"x_ros\"},{\"parameter\":\"Y-Axis\",\"signalID\":28495,\"signalName\":\"y_ros\"}],\"seriesID\":382}],\"subplotID\":1}]}}"
  Robot Simulator : mobileRoboticsTrainingLib/Robot Simulator  Priority=99  Commented=on  mapVar=[]  startX=currentPose(1)  startY=currentPose(2)  startTheta=currentPose(3)  axleLength=L  wheelR=r
  Scope1 : Scope  NumInputPorts=3
  Subscribe1 : ros2lib/Subscribe  topicSource=Select from ROS network  topic=/demo/odom  messageType=nav_msgs/Odometry  sampleTime=-1  QOSHistory=Keep last  QOSDepth=1  QOSReliability=Reliable  QOSDurability=Volatile
      settings: SourceProductBaseCode=RR
  Subscribe2 : ros2lib/Subscribe  topicSource=Select from ROS network  topic=/gps_rasoc/pos  messageType=sensor_msgs/NavSatFix  sampleTime=-1  QOSHistory=Keep last  QOSDepth=1  QOSReliability=Reliable  QOSDurability=Volatile
      settings: SourceProductBaseCode=RR
  Subscribe3 : ros2lib/Subscribe  topicSource=Select from ROS network  topic=/demo/lidar/out  messageType=sensor_msgs/LaserScan  sampleTime=-1  QOSHistory=Keep last  QOSDepth=1  QOSReliability=Reliable  QOSDurability=Volatile
      settings: SourceProductBaseCode=RR
  Subscribe4 : ros2lib/Subscribe  topicSource=Select from ROS network  topic=/gps_rasoc/rasoc_gps/vel  messageType=geometry_msgs/Vector3Stamped  sampleTime=-1  QOSHistory=Keep last  QOSDepth=1  QOSReliability=Reliable  QOSDurability=Volatile
      settings: SourceProductBaseCode=RR
  Subscribe5 : ros2lib/Subscribe  topicSource=Select from ROS network  topic=/imu  messageType=sensor_msgs/Imu  sampleTime=-1  QOSHistory=Keep last  QOSDepth=1  QOSReliability=Reliable  QOSDurability=Volatile
      settings: SourceProductBaseCode=RR
  Subscribe6 : ros2lib/Subscribe  topicSource=Select from ROS network  topic=/gps_base/pos  messageType=sensor_msgs/NavSatFix  sampleTime=-1  QOSHistory=Keep last  QOSDepth=1  QOSReliability=Reliable  QOSDurability=Volatile
      settings: SourceProductBaseCode=RR
  Subsystem : Subsystem  Commented=on
  Sum : Sum  Inputs=-+|
  Sum1 : Sum  Inputs=|+-
  Sum2 : Sum  Inputs=-+|
  Sum3 : Sum  Inputs=-+|
  Terminator : Terminator
  To Workspace2 : ToWorkspace  VariableName=Pose_ros  SampleTime=-1
  XY ROS : simulink/Sinks/XY Graph  xmin=0  xmax=50  ymin=-5  ymax=45  st=-1
  theta-Imu vs Odom : Scope  NumInputPorts=2
  theta_ros : Merge
  v-Gps vs Odom vs Imu : Scope  NumInputPorts=3
  v_ros : Merge
  vw cons vs ros : Scope  NumInputPorts=4
  vw ros : Scope  NumInputPorts=2
  vw2wLwR : Subsystem
  w-Gps vs Odom vs Imu : Scope  NumInputPorts=3
  wLwR ros : Scope  NumInputPorts=2
  w_ros : Merge
  x-Gps vs Odom : Scope  NumInputPorts=2
  x_ros : Merge
  y-Gps vs Odom : Scope  NumInputPorts=2
  y_ros : Merge
  Ranges : Outport
  Angles : Outport  Port=2
  Pose_ros : Outport  Port=3
  wL_ros : Outport  Port=4
  wR_ros : Outport  Port=5
  NewMsg : Outport  Port=6
  tag scope: v_ros=global, w_ros=global
  wires:
  Subscribe1/1 -> NewMsg/1  "odom"
  Subscribe3/1 -> Terminator/1
  Subscribe4/1 -> DGPS Vel/Enable
  Subscribe4/2 -> DGPS Vel/1(In1)
  Subscribe2/1 -> DGPS Position/Enable, [GPS_msg]
  Subscribe2/2 -> DGPS Position/1(In2)
  Subscribe5/1 -> [IMU_msg], IMU/Enable
  Subscribe5/2 -> IMU/1(In2)
  IMU/1(theta_imu) -> [theta_imu]  "theta_imu"
  Subscribe3/2 -> LIDAR/1(In1)
  LIDAR/1(Ranges) -> Ranges/1
  LIDAR/2(Angles) -> Angles/1
  Odometry/1(x_odom) -> [x_odom]
  Odometry/2(y_odom) -> [y_odom]
  Subscribe1/2 -> Odometry/1(In1)
  IMU/2(w_imu) -> [w_imu]  "w_imu"
  IMU/3(v_imu) -> [v_imu]  "v_imu"
  x_ros/1 -> Scope1/1, Record/1, XY ROS/1, MATLAB Function1/1, Mux/1  "x_ros"
  If/1 -> GPS2ROS/Action
  ODOM2ROS/2(y_ros) -> y_ros/2
  GPS2ROS/1(x_ros) -> x_ros/1
  GPS2ROS/2(y_ros) -> y_ros/1
  ODOM2ROS/1(x_ros) -> x_ros/2
  If/2 -> ODOM2ROS/Action
  y_ros/1 -> Mux/2, MATLAB Function1/2, Record/2, XY ROS/2  "y_ros"
  [x_gps] -> Scope1/2, GPS2ROS/1(x_gps)  "xg_GPS"
  [y_gps] -> GPS2ROS/2(y_gps)
  [x_odom] -> Scope1/3, ODOM2ROS/1(x_odom)  "xg_odom"
  [y_odom] -> ODOM2ROS/2(y_odom)
  [theta_odom] -> ODOM2ROS_theta/1(theta_odom)
  [theta_imu] -> IMU2ROS/1(theta_imu)
  If1/2 -> ODOM2ROS_theta/Action
  ODOM2ROS_theta/1(theta_ros) -> theta_ros/2
  IMU2ROS/1(theta_ros) -> theta_ros/1
  If1/1 -> IMU2ROS/Action
  theta_ros/1 -> MATLAB Function1/3, Mux/3
  Odometry/3(theta_odom) -> [theta_odom]
  Constant/1 -> MATLAB Function/5(a)
  MATLAB Function/1(v) -> Moving Average/1  "v_gps"
  MATLAB Function/2(w) -> [w_gps]  "w_gps"
  vw2wLwR/2(wR_ros) -> Subsystem/2(wr), wLwR ros/2, wR_ros/1  "wR_ros"
  vw2wLwR/1(wL_ros) -> wLwR ros/1, Subsystem/1(wl), wL_ros/1  "wL_ros"
  Mux/1 -> To Workspace2/1, Pose_ros/1
  [w_gps] -> GPS2ROS/4(w_gps)
  [v_gps] -> GPS2ROS/3(v_gps)
  w_ros/1 -> vw2wLwR/2(w_ros), vw ros/2, [w_ros]  "w_ros"
  Odometry/4(v_odom) -> [v_odom]
  Odometry/5(w_odom) -> [w_odom]
  DGPS Vel/1(dx_gps) -> MATLAB Function/1(dx)  "dx_gps"
  DGPS Vel/2(dy_gps) -> MATLAB Function/2(dy)  "dy_gps"
  [GPS_msg] -> If/1
  [IMU_msg] -> If1/1
  Subscribe6/2 -> DGPS Base Position/1(In2)
  Subscribe6/1 -> DGPS Base Position/Enable
  Constant1/1 -> Sum/1
  Sum/1 -> Abs/1
  Constant2/1 -> Sum1/2
  Sum1/1 -> Abs1/1
  DGPS Position/1(x_gps) -> Sum3/1, x-Gps vs Odom/1, [x_gps]  "x_gps"
  DGPS Position/2(y_gps) -> Sum2/1, y-Gps vs Odom/1, [y_gps]  "y_gps"
  Sum3/1 -> Error gps/1  "e_x"
  Sum2/1 -> Error gps/2  "e_y"
  [x_odom] -> x-Gps vs Odom/2, Sum3/2  "x_odom"
  [y_odom] -> y-Gps vs Odom/2, Sum2/2  "y_odom"
  DGPS Base Position/2(yb_gps) -> Pos base gps/2, Sum1/1  "yb_gps"
  DGPS Base Position/1(xb_gps) -> Sum/2, Pos base gps/1  "xb_gps"
  [w_odom] -> w-Gps vs Odom vs Imu/2
  [w_imu] -> w-Gps vs Odom vs Imu/3
  [w_gps] -> w-Gps vs Odom vs Imu/1
  [theta_imu] -> theta-Imu vs Odom/1
  [theta_imu] -> MATLAB Function/3(theta)
  [theta_odom] -> theta-Imu vs Odom/2
  [v_odom] -> v-Gps vs Odom vs Imu/2
  [v_imu] -> v-Gps vs Odom vs Imu/3
  [v_gps] -> v-Gps vs Odom vs Imu/1
  [w_imu] -> MATLAB Function/4(dtheta)
  Moving Average/1 -> [v_gps]  "v_gps"
  [v_odom] -> ODOM2ROS/3(v_odom)
  [w_odom] -> ODOM2ROS/4(w_odom)
  GPS2ROS/3(v_ros) -> v_ros/1
  ODOM2ROS/3(v_ros) -> v_ros/2
  GPS2ROS/4(w_ros) -> w_ros/1
  ODOM2ROS/4(w_ros) -> w_ros/2
  Abs/1 -> Errpr base gps/1  "e_xb"
  Abs1/1 -> Errpr base gps/2  "e_yb"
  v_ros/1 -> [v_ros], vw ros/1, vw2wLwR/1(v_ros)  "v_ros"
  [w_ros] -> vw cons vs ros/3
  [v_ros] -> vw cons vs ros/1
  [v_cons] -> vw cons vs ros/2
  [w_cons] -> vw cons vs ros/4
  Constant3/1 -> MATLAB Function1/4
